simulink library "motohawk_engine_lib"  (Simulink 6.3)
undefined symbols (not defined in the file or in its folder): cast_val, IndPowerMax, InjSequence, lookup_group, MAF_Sensor_p, motohawk_tex, motohawk_vardec_config_group, motohawk_vardec_path, SampleTime, SparkSequence, SteadyStateECT, txtTitle, WarmUpTimeConst
libraries: MotoHawk_lib x234, motohawk_annotations_lib x22, motohawk_control_primitives_lib x20, motohawk_engine_lib x8, motohawk_control_primitives_lib_new x3
(part 5 of 7)

== system motohawk_engine_lib/PWM Characterization ==
  note: The outputs of this block are designed to be
      | directly connected to a MotoHawk PWM block.
  EngUnits : Inport
  Convert to integer 0.01Hz resolution : Gain  Gain=100  SaturateOnIntegerOverflow=on
  Convert to integer 14-bit PWM resolution : Gain  Gain=40.95  SaturateOnIntegerOverflow=on
  Data Type Conversion1 : DataTypeConversion  SaturateOnIntegerOverflow=on  RndMeth=Zero
  Data Type Conversion2 : DataTypeConversion  OutDataTypeMode=uint32  SaturateOnIntegerOverflow=on  RndMeth=Zero
  Data Type Conversion3 : DataTypeConversion  OutDataTypeMode=int16  SaturateOnIntegerOverflow=on  RndMeth=Zero
  Product : Product  SaturateOnIntegerOverflow=on  InputSameDT=on
  Saturation : motohawk_control_primitives_lib/Saturation
  Sum : Sum  Inputs=|++  SaturateOnIntegerOverflow=on
  motohawk_calibration : MotoHawk_lib/Calibration & Probing Blocks/motohawk_calibration  nam=[prefix 'Gain']  val=1  storage=Calibration  show_more=on  name_source=Use Parameter  data_type=double  read_level=1  write_level=1  ovr_cals=on  view_as=Number  enum_struct={'Disabled', 'Enabled'}  vector_style=Wide Row  use_help_units=on  help='Scaling from engineering units to PWM duty cycle'  units=['%/' units]  use_header_enum=off  row_header_enum={}  col_header_enum={}  use_min_max=off  min_val=-inf  max_val=inf  use_precision=off  precision=''  gain=1  offset=0  exp=1  use_mototune_group=on  mototune_group=[group ' | ' nam ' Config']
  motohawk_calibration1 : MotoHawk_lib/Calibration & Probing Blocks/motohawk_calibration  nam=[prefix 'Offset']  val=0  storage=Calibration  show_more=on  name_source=Use Parameter  data_type=double  read_level=1  write_level=1  ovr_cals=on  view_as=Number  enum_struct={'Disabled', 'Enabled'}  vector_style=Wide Row  use_help_units=on  help='Offset from engineering units to PWM duty cycle'  units='%'  use_header_enum=off  row_header_enum={}  col_header_enum={}  use_min_max=off  min_val=-inf  max_val=inf  use_precision=off  precision=''  gain=1  offset=0  exp=1  use_mototune_group=on  mototune_group=[group ' | ' nam ' Config']
  motohawk_calibration2 : MotoHawk_lib/Calibration & Probing Blocks/motohawk_calibration  nam=[prefix 'MinLimit']  val=0  storage=Calibration  show_more=on  name_source=Use Parameter  data_type=double  read_level=1  write_level=1  ovr_cals=on  view_as=Number  enum_struct={'Disabled', 'Enabled'}  vector_style=Wide Row  use_help_units=on  help='Minimum limit of PWM signal.'  units='%'  use_header_enum=off  row_header_enum={}  col_header_enum={}  use_min_max=off  min_val=-inf  max_val=inf  use_precision=off  precision=''  gain=1  offset=0  exp=1  use_mototune_group=on  mototune_group=[group ' | ' nam ' Config']
  motohawk_calibration3 : MotoHawk_lib/Calibration & Probing Blocks/motohawk_calibration  nam=[prefix 'MaxLimit']  val=100  storage=Calibration  show_more=on  name_source=Use Parameter  data_type=double  read_level=1  write_level=1  ovr_cals=on  view_as=Number  enum_struct={'Disabled', 'Enabled'}  vector_style=Wide Row  use_help_units=on  help='Maximum limit of PWM signal.'  units='%'  use_header_enum=off  row_header_enum={}  col_header_enum={}  use_min_max=off  min_val=-inf  max_val=inf  use_precision=off  precision=''  gain=1  offset=0  exp=1  use_mototune_group=on  mototune_group=[group ' | ' nam ' Config']
  motohawk_calibration4 : MotoHawk_lib/Calibration & Probing Blocks/motohawk_calibration  nam=[prefix 'Frequency']  val=100  storage=Calibration  show_more=on  name_source=Use Parameter  data_type=double  read_level=1  write_level=1  ovr_cals=on  view_as=Number  enum_struct={'Disabled', 'Enabled'}  vector_style=Wide Row  use_help_units=on  help='Frequency of PWM output'  units='Hz'  use_header_enum=off  row_header_enum={}  col_header_enum={}  use_min_max=off  min_val=-inf  max_val=inf  use_precision=off  precision=''  gain=1  offset=0  exp=1  use_mototune_group=on  mototune_group=[group ' | ' nam ' Config']
  motohawk_override_abs2 : MotoHawk_lib/Calibration & Probing Blocks/motohawk_override_abs  parent_name=nam  show_more=on  name_source=Use Parameter  parent_read_level=1  parent_override_level=1  view_as=Number  enum_struct={'Disabled', 'Enabled'}  use_help_units=on  parent_help='Override result of linear sensor characterization, in engineering units'  parent_units=units  use_min_max=on  parent_min=-inf  parent_max=inf  use_precision=off  parent_precision=''  parent_gain=1  parent_offset=0  parent_exp=1  use_mototune_group=on  parent_group=group
  motohawk_probe2 : MotoHawk_lib/Calibration & Probing Blocks/motohawk_probe  nam=[prefix 'DutyCycle']  show_more=on  name_source=Use Parameter  read_level=1  view_as=Number  enum_struct={'Disabled', 'Enabled'}  vector_style=Wide Row  use_help_units=on  help='Actual duty cycle of actuator'  units='%'  use_header_enum=off  row_header_enum={}  col_header_enum={}  use_precision=off  precision=''  gain=1  offset=0  exp=1  use_mototune_group=on  mototune_group=group
  DutyCycle : Outport
  Frequency : Outport  Port=2
  wires:
  Data Type Conversion2/1 -> Frequency/1
  Convert to integer 0.01Hz resolution/1 -> Data Type Conversion2/1
  motohawk_calibration4/1 -> Convert to integer 0.01Hz resolution/1
  Data Type Conversion1/1 -> Product/1
  motohawk_override_abs2/1 -> Data Type Conversion1/1
  EngUnits/1 -> motohawk_override_abs2/1
  Product/1 -> Sum/1
  motohawk_calibration1/1 -> Sum/2
  motohawk_calibration/1 -> Product/2
  Data Type Conversion3/1 -> DutyCycle/1
  Convert to integer 14-bit PWM resolution/1 -> Data Type Conversion3/1
  Sum/1 -> Saturation/1
  Saturation/1 -> Convert to integer 14-bit PWM resolution/1, motohawk_probe2/1
  motohawk_calibration2/1 -> Saturation/2
  motohawk_calibration3/1 -> Saturation/3

== system motohawk_engine_lib/Spark Coil Characterization ==
  SparkEnergy [mJ] : Inport
  SysVolt10Idx : Inport  Port=2
  Constant : Constant  Value=1000
  Constant1 : Constant  Value=0
  Only Enable Spark when Energy is Above Zero : RelationalOperator  Operator=>  ZeroCross=off  InputSameDT=on
  Product : Product  Inputs=*/  SaturateOnIntegerOverflow=on
  Sum : Sum  Inputs=|++  SaturateOnIntegerOverflow=on
  motohawk_TitleBlock : motohawk_annotations_lib/motohawk_TitleBlock  BlockType_='Mototron_Title_Block'  ttl='Spark Coil Characterization\newline\rmCalculations for spark coil dwell time vs. desired spark energy'  copyright="'THE INFORMATION CONTAINED IN THIS\\newlineDRAWING IS THE SOLE PROPERTY OF\\newlineMOTOTRON.  ANY REPRODUCTION IN\\newline PART OR AS A WHOLE WITHOUT THE\\newlineWRITTEN PERMISSION OF MOTOTRON\\newline IS PROHIBITED.\\fontsize{16}\\rm\\copyright\\rm\\fontsize{10} 2005'"  address='\fontsize{22}\it\fontname{Arial Black}MotoTron Corporation \fontname{Arial}\fontsize{10}\newline505 Marion Road, Oshkosh, WI, 54901\newlinewww.mototron.com (734) 822-7700'  image_file='mh.jpg'  pretty_print=on  edit_text=[motohawk_tex(get_param(bdroot, 'Description')) '\rm\newline' motohawk_tex(get_param(gcs, 'Name'))]  edit_as=6
  motohawk_calibration : MotoHawk_lib/Calibration & Probing Blocks/motohawk_calibration  nam='CoilDrvrDlyTime'  val=CoilDrvrDlyTime  storage=Calibration  show_more=on  name_source=Use Parameter  data_type=Inherit from 'Default Value'  read_level=1  write_level=1  ovr_cals=on  view_as=Number  enum_struct={'Disabled', 'Enabled'}  vector_style=Wide Row  use_help_units=on  help='Spark Coil Driver Delay Time'  units='us'  use_header_enum=off  row_header_enum={}  col_header_enum={}  use_min_max=off  min_val=-inf  max_val=inf  use_precision=off  precision=''  gain=1  offset=0  exp=1  use_mototune_group=off  mototune_group=lookup_group(gcb, 'CoilDrvrDlyTime')
  motohawk_interpolation_2d : MotoHawk_lib/Lookup Tables/motohawk_interpolation_2d  nam='CoilDwell'  table_data=CoilDwellMap  show_more=on  data_type=Inherit from 'Table Data'  storage=NonAdaptive  read_level=1  write_level=1  ovr_cals=on  use_help=on  help='Spark dwell time'  units='ms'  use_min_max=off  min_val=-inf  max_val=inf  use_precision=off  precision=''  gain=1  offset=0  exp=1  use_links=on  row_prelookup_block=''  col_prelookup_block=''  output_name='CoilDwell'  use_mototune_group=off  mototune_group=lookup_group(gcb, 'CoilDwell')
  motohawk_prelookup1 : MotoHawk_lib/Lookup Tables/motohawk_prelookup  nam='SpkEnergy10'  breakpoint_data=SpkEnergy10IdxArr  show_more=on  data_type=Inherit from 'Table Data'  storage=Constant  read_level=1  write_level=1  ovr_cals=on  use_help=on  help='Prelookup for Spark Energy'  units='mJ'  use_min_max=off  min_val=-inf  max_val=inf  use_precision=off  precision=''  gain=1  offset=0  exp=1  use_links=on  input_name='SparkEnergy'  use_mototune_group=off  mototune_group=lookup_group(gcb, 'SpkEnergy10')
  motohawk_probe : MotoHawk_lib/Calibration & Probing Blocks/motohawk_probe  nam='CoilDwell'  show_more=on  name_source=Use Parameter  read_level=1  view_as=Number  enum_struct={'Disabled', 'Enabled'}  vector_style=Wide Row  use_help_units=on  help='Total electrical spark dwell time'  units='ms'  use_header_enum=off  row_header_enum={}  col_header_enum={}  use_precision=off  precision=''  gain=1  offset=0  exp=1  use_mototune_group=off  mototune_group=lookup_group(gcb, 'CoilDwell')
  motohawk_probe1 : MotoHawk_lib/Calibration & Probing Blocks/motohawk_probe  nam='SparkEnergy'  show_more=on  name_source=Use Parameter  read_level=1  view_as=Number  enum_struct={'Disabled', 'Enabled'}  vector_style=Wide Row  use_help_units=on  help='Commanded spark energy, before conversion to dwell time'  units='mJ'  use_header_enum=off  row_header_enum={}  col_header_enum={}  use_precision=off  precision=''  gain=1  offset=0  exp=1  use_mototune_group=off  mototune_group=lookup_group(gcb, 'SparkEnergy')
  SparkDwell [ms] : Outport
  SparkEnable [bool] : Outport  Port=2
  wires:
  Constant1/1 -> Only Enable Spark when Energy is Above Zero/2
  Only Enable Spark when Energy is Above Zero/1 -> SparkEnable [bool]/1
  Constant/1 -> Product/2
  Product/1 -> Sum/2
  motohawk_calibration/1 -> Product/1
  motohawk_interpolation_2d/1 -> Sum/1
  Sum/1 -> SparkDwell [ms]/1, motohawk_probe/1
  SparkEnergy [mJ]/1 -> Only Enable Spark when Energy is Above Zero/1, motohawk_probe1/1, motohawk_prelookup1/1
  motohawk_prelookup1/1 -> motohawk_interpolation_2d/1  "SpkEnergy10Idx"
  SysVolt10Idx/1 -> motohawk_interpolation_2d/2  "SysVolt10Idx"

== system motohawk_engine_lib/Spark Coil Output ==
  SparkEnable : Inport
  SparkStartAngle [degCA] : Inport  Port=2
  SparkStopAngle [degCA] : Inport  Port=3
  CylEnable : Inport  Port=4
  Data Type Conversion : DataTypeConversion  SaturateOnIntegerOverflow=on  RndMeth=Zero
  Data Type Conversion1 : DataTypeConversion  SaturateOnIntegerOverflow=on  RndMeth=Zero
  Data Type Conversion2 : DataTypeConversion  SaturateOnIntegerOverflow=on  RndMeth=Zero
  Gain1 : Gain  Gain=16  SaturateOnIntegerOverflow=on
  Gain2 : Gain  Gain=16  SaturateOnIntegerOverflow=on
  Logical Operator : Logic  AllPortsSameDT=off
  motohawk_seq_out_est : MotoHawk_lib/Advanced Digital I//O/motohawk_seq_out_est  text_resource=EST 1  code_resource=RES_EST1  val_resource=-1  target=ECU555_80  resource_enum_str=(None)=-1,EST 1=36,EST 2=37,EST 3=38,EST 4=39,EST 5=40,EST 6=41,EST 7=42,EST 8=43,EST 9=44,EST 10=45,EST 11=46,EST 12=47,EST 13=48,EST 14=49,EST 15=50,EST 16=51  pulse_number=0  pulse_angle_offset=offset  stop_mode=Angle Controlled  update_mode=OS  granularity=Fine  use_max_duration=off  use_vardec=off  nam='EST'  read_level=1  write_level=1  group='System | I/O Pins | Outputs Config'
  wires:
  Gain2/1 -> Data Type Conversion1/1
  Gain1/1 -> Data Type Conversion2/1
  SparkStartAngle [degCA]/1 -> Gain2/1
  SparkStopAngle [degCA]/1 -> Gain1/1
  Data Type Conversion/1 -> motohawk_seq_out_est/1
  Data Type Conversion1/1 -> motohawk_seq_out_est/2
  Data Type Conversion2/1 -> motohawk_seq_out_est/3
  Logical Operator/1 -> Data Type Conversion/1
  SparkEnable/1 -> Logical Operator/2
  CylEnable/1 -> Logical Operator/1

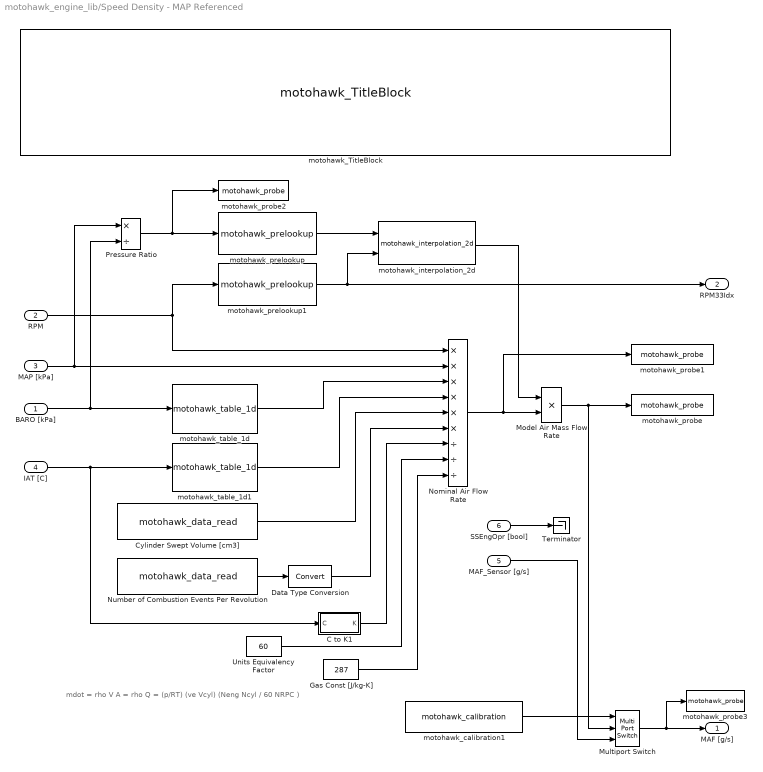
== system motohawk_engine_lib/Speed Density - MAP Referenced ==
  note: mdot = rho V A = rho Q = (p/RT) (ve Vcyl) (Neng Ncyl / 60 NRPC )
  BARO [kPa] : Inport
  RPM : Inport  Port=2
  MAP [kPa] : Inport  Port=3
  IAT [C] : Inport  Port=4
  MAF_Sensor [g/s] : Inport  Port=5
  SSEngOpr [bool] : Inport  Port=6
  C to K1 : Subsystem
      mask Display: disp('to')
  Cylinder Swept Volume [cm3] : MotoHawk_lib/Data Storage Blocks/motohawk_data_read  source=Lookup By Name  structure=Scalar  operation=Read scalar from location by index  sz_vec=-1  sz_row=-1  sz_col=-1  typ=double  nam='CylSweptVol'  checkNull=on  struct_inst_name='Struct1'
  Data Type Conversion : DataTypeConversion  SaturateOnIntegerOverflow=on  RndMeth=Zero
  Gas Const [J/kg-K] : Constant  Value=287
  Model Air Mass Flow Rate : Product  Inputs=**  SaturateOnIntegerOverflow=on  InputSameDT=on
  Multiport Switch : MultiPortSwitch  Inputs=2  zeroidx=on  SaturateOnIntegerOverflow=on  InputSameDT=on
  Nominal Air Flow Rate : Product  Inputs=******///  SaturateOnIntegerOverflow=on  InputSameDT=on
  Number of Combustion Events Per Revolution : MotoHawk_lib/Data Storage Blocks/motohawk_data_read  source=Lookup By Name  structure=Scalar  operation=Read scalar from location by index  sz_vec=-1  sz_row=-1  sz_col=-1  typ=uint8  nam='CombEventsPerRev'  checkNull=on  struct_inst_name='Struct1'
  Pressure Ratio : Product  Inputs=*/  SaturateOnIntegerOverflow=on  InputSameDT=on
  Terminator : Terminator
  Units Equivalency Factor : Constant  Value=60
  motohawk_TitleBlock : motohawk_annotations_lib/motohawk_TitleBlock  BlockType_='Mototron_Title_Block'  ttl='Compute Mass Airflow from Manifold Pressure and Temperature\newline\rmUses a Volumetric Efficiency map to adjust the results of the ideal gas law.'  copyright="'THE INFORMATION CONTAINED IN THIS\\newlineDRAWING IS THE SOLE PROPERTY OF\\newlineMOTOTRON.  ANY REPRODUCTION IN\\newline PART OR AS A WHOLE WITHOUT THE\\newlineWRITTEN PERMISSION OF MOTOTRON\\newline IS PROHIBITED.\\fontsize{16}\\rm\\copyright\\rm\\fontsize{10} 2005'"  address='\fontsize{22}\it\fontname{Arial Black}MotoTron Corporation \fontname{Arial}\fontsize{10}\newline505 Marion Road, Oshkosh, WI, 54901\newlinewww.mototron.com (734) 822-7700'  image_file='mh.jpg'  pretty_print=on  edit_text=[motohawk_tex(get_param(bdroot, 'Description')) '\rm\newline' motohawk_tex(get_param(gcs, 'Name'))]  edit_as=6
  motohawk_calibration1 : MotoHawk_lib/Calibration & Probing Blocks/motohawk_calibration  nam='MAF_Source'  val=MAF_Source  storage=Calibration  show_more=on  name_source=Use Parameter  data_type=uint8  read_level=1  write_level=1  ovr_cals=on  view_as=Enumeration  enum_struct={'Model from MAP', 'Use MAF sensor directly'}  vector_style=Wide Row  use_help_units=on  help='Selects the source for the fueling algorithm'  units=''  use_header_enum=off  row_header_enum={}  col_header_enum={}  use_min_max=off  min_val=-inf  max_val=inf  use_precision=off  precision=''  gain=1  offset=0  exp=1  use_mototune_group=on  mototune_group=lookup_group(gcb)
  motohawk_interpolation_2d : MotoHawk_lib/Lookup Tables/motohawk_interpolation_2d  nam='VolEff'  table_data=VolEffMap  show_more=on  data_type=Inherit from 'Table Data'  storage=NonAdaptive  read_level=1  write_level=1  ovr_cals=on  use_help=on  help='Volumetric Efficiency'  units='mult'  use_min_max=off  min_val=-inf  max_val=inf  use_precision=on  precision='6.4'  gain=1  offset=0  exp=1  use_links=off  row_prelookup_block=''  col_prelookup_block=''  output_name=''  use_mototune_group=on  mototune_group=lookup_group(gcb)
  motohawk_prelookup : MotoHawk_lib/Lookup Tables/motohawk_prelookup  nam='PressRatio17'  breakpoint_data=PressRatio17IdxArr  show_more=on  data_type=Inherit from 'Table Data'  storage=Constant  read_level=1  write_level=1  ovr_cals=on  use_help=on  help='Prelookup for Pressure Ratio'  units='ratio'  use_min_max=off  min_val=-inf  max_val=inf  use_precision=off  precision=''  gain=1  offset=0  exp=1  use_links=on  input_name='PressRatio'  use_mototune_group=on  mototune_group=lookup_group(gcb)
  motohawk_prelookup1 : MotoHawk_lib/Lookup Tables/motohawk_prelookup  nam='RPM17'  breakpoint_data=RPM17IdxArr  show_more=on  data_type=Inherit from 'Table Data'  storage=Constant  read_level=1  write_level=1  ovr_cals=on  use_help=on  help='Prelookup for RPM'  units='RPM'  use_min_max=off  min_val=-inf  max_val=inf  use_precision=off  precision=''  gain=1  offset=0  exp=1  use_links=on  input_name='RPM'  use_mototune_group=on  mototune_group=lookup_group(gcb)
  motohawk_probe : MotoHawk_lib/Calibration & Probing Blocks/motohawk_probe  nam='MAF_Model'  show_more=on  name_source=Use Parameter  read_level=1  view_as=Number  enum_struct={'Disabled', 'Enabled'}  vector_style=Wide Row  use_help_units=on  help='Air Mass Flow Rate - Port Total'  units='g/s'  use_header_enum=off  row_header_enum={}  col_header_enum={}  use_precision=off  precision=''  gain=1  offset=0  exp=1  use_mototune_group=on  mototune_group=lookup_group(gcb)
  motohawk_probe1 : MotoHawk_lib/Calibration & Probing Blocks/motohawk_probe  nam='MAF_Ideal'  show_more=on  name_source=Use Parameter  read_level=1  view_as=Number  enum_struct={'Disabled', 'Enabled'}  vector_style=Wide Row  use_help_units=on  help='Air Mass Flow Rate - ideal'  units='g/s'  use_header_enum=off  row_header_enum={}  col_header_enum={}  use_precision=off  precision=''  gain=1  offset=0  exp=1  use_mototune_group=on  mototune_group=lookup_group(gcb)
  motohawk_probe2 : MotoHawk_lib/Calibration & Probing Blocks/motohawk_probe  nam='PressRatio'  show_more=on  name_source=Use Parameter  read_level=1  view_as=Number  enum_struct={'Disabled', 'Enabled'}  vector_style=Wide Row  use_help_units=on  help='Pressure ratio - MAP over BARO'  units='ratio'  use_header_enum=off  row_header_enum={}  col_header_enum={}  use_precision=off  precision=''  gain=1  offset=0  exp=1  use_mototune_group=on  mototune_group=lookup_group(gcb)
  motohawk_probe3 : MotoHawk_lib/Calibration & Probing Blocks/motohawk_probe  nam='MAF'  show_more=on  name_source=Use Parameter  read_level=1  view_as=Number  enum_struct={'Disabled', 'Enabled'}  vector_style=Wide Row  use_help_units=on  help='Air mass flow rate at the intake manifold - Used by the fueling algorithm'  units='g/s'  use_header_enum=off  row_header_enum={}  col_header_enum={}  use_precision=off  precision=''  gain=1  offset=0  exp=1  use_mototune_group=on  mototune_group=lookup_group(gcb)
  motohawk_table_1d : MotoHawk_lib/Lookup Tables/motohawk_table_1d  nam='VEPressCorr'  bp_nam='BARO17'  breakpoint_data=BARO17IdxArr  table_data=VEPressCorrTbl  show_more=on  bp_data_type=Inherit from 'Breakpoint Data'  table_data_type=Inherit from 'Table Data'  storage=NonAdaptive  read_level=1  write_level=1  ovr_cals=on  use_help=off  help=''  bp_units=''  table_units=''  use_min_max=off  bp_min_val=-inf  bp_max_val=inf  min_val=-inf  max_val=inf  use_precision=off  use_breakpoint=off  b_precision=''  b_gain=1  b_offset=0  b_exp=1  use_table=off  t_precision=''  t_gain=1  t_offset=0  t_exp=1  use_links=on  input_name='BARO'  output_name=''  use_mototune_group=on  mototune_group=lookup_group(gcb)
  motohawk_table_1d1 : MotoHawk_lib/Lookup Tables/motohawk_table_1d  nam='VETempCorr'  bp_nam='IAT17'  breakpoint_data=IAT17IdxArr  table_data=VETempCorrTbl  show_more=on  bp_data_type=Inherit from 'Breakpoint Data'  table_data_type=Inherit from 'Table Data'  storage=NonAdaptive  read_level=1  write_level=1  ovr_cals=on  use_help=off  help=''  bp_units=''  table_units=''  use_min_max=off  bp_min_val=-inf  bp_max_val=inf  min_val=-inf  max_val=inf  use_precision=off  use_breakpoint=off  b_precision=''  b_gain=1  b_offset=0  b_exp=1  use_table=off  t_precision=''  t_gain=1  t_offset=0  t_exp=1  use_links=on  input_name='IAT'  output_name=''  use_mototune_group=on  mototune_group=lookup_group(gcb)
  MAF [g/s] : Outport
  RPM33Idx : Outport  Port=2
  wires:
  SSEngOpr [bool]/1 -> Terminator/1
  Data Type Conversion/1 -> Nominal Air Flow Rate/6
  Nominal Air Flow Rate/1 -> motohawk_probe1/1, Model Air Mass Flow Rate/2
  Gas Const [J/kg-K]/1 -> Nominal Air Flow Rate/9
  Units Equivalency Factor/1 -> Nominal Air Flow Rate/8
  C to K1/1(K) -> Nominal Air Flow Rate/7
  Number of Combustion Events Per Revolution/1 -> Data Type Conversion/1
  Cylinder Swept Volume [cm3]/1 -> Nominal Air Flow Rate/5
  motohawk_table_1d1/1 -> Nominal Air Flow Rate/4
  motohawk_table_1d/1 -> Nominal Air Flow Rate/3
  MAP [kPa]/1 -> Nominal Air Flow Rate/2, Pressure Ratio/1
  BARO [kPa]/1 -> motohawk_table_1d/1, Pressure Ratio/2
  RPM/1 -> motohawk_prelookup1/1, Nominal Air Flow Rate/1
  IAT [C]/1 -> motohawk_table_1d1/1, C to K1/1(C)
  Pressure Ratio/1 -> motohawk_probe2/1, motohawk_prelookup/1
  Model Air Mass Flow Rate/1 -> Multiport Switch/2, motohawk_probe/1
  motohawk_interpolation_2d/1 -> Model Air Mass Flow Rate/1
  motohawk_prelookup/1 -> motohawk_interpolation_2d/1
  motohawk_prelookup1/1 -> motohawk_interpolation_2d/2, RPM33Idx/1
  MAF_Sensor [g/s]/1 -> Multiport Switch/3
  Multiport Switch/1 -> MAF [g/s]/1, motohawk_probe3/1
  motohawk_calibration1/1 -> Multiport Switch/1

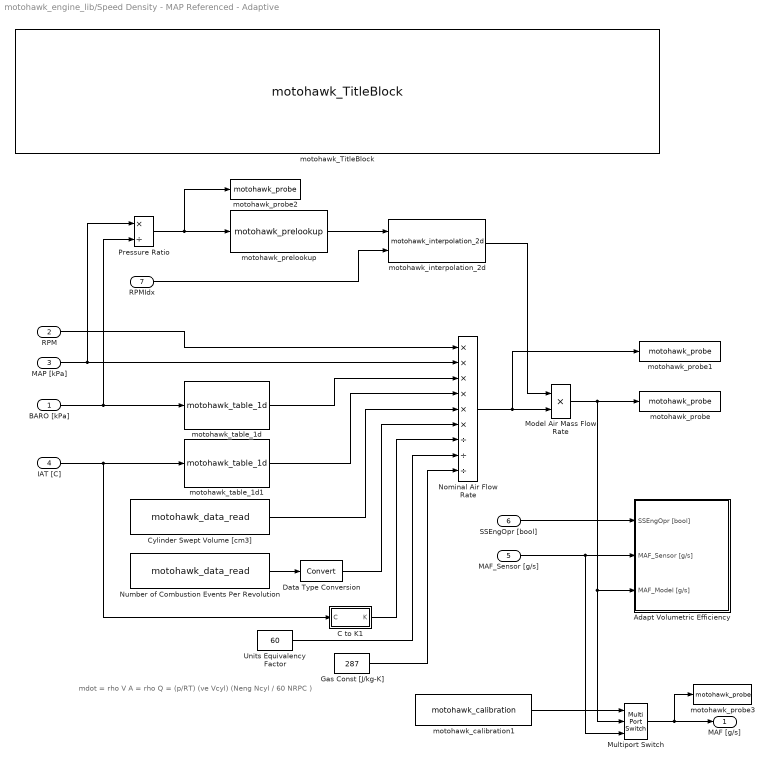
== system motohawk_engine_lib/Speed Density - MAP Referenced - Adaptive ==
  note: mdot = rho V A = rho Q = (p/RT) (ve Vcyl) (Neng Ncyl / 60 NRPC )
  BARO [kPa] : Inport
  RPM : Inport  Port=2
  MAP [kPa] : Inport  Port=3
  IAT [C] : Inport  Port=4
  MAF_Sensor [g/s] : Inport  Port=5
  SSEngOpr [bool] : Inport  Port=6
  RPMIdx : Inport  Port=7
  Adapt Volumetric Efficiency : Subsystem
  C to K1 : Subsystem
      mask Display: disp('to')
  Cylinder Swept Volume [cm3] : MotoHawk_lib/Data Storage Blocks/motohawk_data_read  source=Lookup By Name  structure=Scalar  operation=Read scalar from location by index  sz_vec=-1  sz_row=-1  sz_col=-1  typ=double  nam='CylSweptVol'  checkNull=on  struct_inst_name='Struct1'
  Data Type Conversion : DataTypeConversion  SaturateOnIntegerOverflow=on  RndMeth=Zero
  Gas Const [J/kg-K] : Constant  Value=287
  Model Air Mass Flow Rate : Product  Inputs=**  SaturateOnIntegerOverflow=on  InputSameDT=on
  Multiport Switch : MultiPortSwitch  Inputs=2  zeroidx=on  SaturateOnIntegerOverflow=on  InputSameDT=on
  Nominal Air Flow Rate : Product  Inputs=******///  SaturateOnIntegerOverflow=on  InputSameDT=on
  Number of Combustion Events Per Revolution : MotoHawk_lib/Data Storage Blocks/motohawk_data_read  source=Lookup By Name  structure=Scalar  operation=Read scalar from location by index  sz_vec=-1  sz_row=-1  sz_col=-1  typ=uint8  nam='CombEventsPerRev'  checkNull=on  struct_inst_name='Struct1'
  Pressure Ratio : Product  Inputs=*/  SaturateOnIntegerOverflow=on  InputSameDT=on
  Units Equivalency Factor : Constant  Value=60
  motohawk_TitleBlock : motohawk_annotations_lib/motohawk_TitleBlock  BlockType_='Mototron_Title_Block'  ttl='Compute Mass Airflow from Manifold Pressure and Temperature\newline\rmUses a Volumetric Efficiency map to adjust the results of the ideal gas law.'  copyright="'THE INFORMATION CONTAINED IN THIS\\newlineDRAWING IS THE SOLE PROPERTY OF\\newlineMOTOTRON.  ANY REPRODUCTION IN\\newline PART OR AS A WHOLE WITHOUT THE\\newlineWRITTEN PERMISSION OF MOTOTRON\\newline IS PROHIBITED.\\fontsize{16}\\rm\\copyright\\rm\\fontsize{10} 2005'"  address='\fontsize{22}\it\fontname{Arial Black}MotoTron Corporation \fontname{Arial}\fontsize{10}\newline505 Marion Road, Oshkosh, WI, 54901\newlinewww.mototron.com (734) 822-7700'  image_file='mh.jpg'  pretty_print=on  edit_text=[motohawk_tex(get_param(bdroot, 'Description')) '\rm\newline' motohawk_tex(get_param(gcs, 'Name'))]  edit_as=6
  motohawk_calibration1 : MotoHawk_lib/Calibration & Probing Blocks/motohawk_calibration  nam='MAF_Source'  val=0  storage=Display  show_more=on  name_source=Use Parameter  data_type=uint8  read_level=1  write_level=1  ovr_cals=on  view_as=Enumeration  enum_struct={'Model from MAP', 'Use MAF sensor directly'}  vector_style=Wide Row  use_help_units=on  help='Selects the source for the fueling algorithm'  units=''  use_header_enum=off  row_header_enum={}  col_header_enum={}  use_min_max=off  min_val=-inf  max_val=inf  use_precision=off  precision=''  gain=1  offset=0  exp=1  use_mototune_group=on  mototune_group=lookup_group(gcb)
  motohawk_interpolation_2d : MotoHawk_lib/Lookup Tables/motohawk_interpolation_2d  nam='VolEff'  table_data=VolEffMap  show_more=on  data_type=Inherit from 'Table Data'  storage=Adaptive - NonVolatile  read_level=1  write_level=1  ovr_cals=on  use_help=off  help='Volumetric Efficiency'  units='mult'  use_min_max=off  min_val=-inf  max_val=inf  use_precision=off  precision='5.3'  gain=1  offset=0  exp=1  use_links=off  row_prelookup_block=''  col_prelookup_block=''  output_name=''  use_mototune_group=off  mototune_group=lookup_group(gcb)
  motohawk_prelookup : MotoHawk_lib/Lookup Tables/motohawk_prelookup  nam='PressRatio17'  breakpoint_data=PressRatio17IdxArr  show_more=on  data_type=Inherit from 'Table Data'  storage=Constant  read_level=1  write_level=1  ovr_cals=on  use_help=on  help='Prelookup for Pressure Ratio'  units='ratio'  use_min_max=off  min_val=-inf  max_val=inf  use_precision=off  precision=''  gain=1  offset=0  exp=1  use_links=on  input_name='PressRatio'  use_mototune_group=on  mototune_group='Indexes'
  motohawk_probe : MotoHawk_lib/Calibration & Probing Blocks/motohawk_probe  nam='MAF_Model'  show_more=on  name_source=Use Parameter  read_level=1  view_as=Number  enum_struct={'Disabled', 'Enabled'}  vector_style=Wide Row  use_help_units=on  help='Air Mass Flow Rate - Port Total'  units='g/s'  use_header_enum=off  row_header_enum={}  col_header_enum={}  use_precision=off  precision=''  gain=1  offset=0  exp=1  use_mototune_group=on  mototune_group=lookup_group(gcb)
  motohawk_probe1 : MotoHawk_lib/Calibration & Probing Blocks/motohawk_probe  nam='MAF_Ideal'  show_more=on  name_source=Use Parameter  read_level=1  view_as=Number  enum_struct={'Disabled', 'Enabled'}  vector_style=Wide Row  use_help_units=on  help='Air Mass Flow Rate - ideal'  units='g/s'  use_header_enum=off  row_header_enum={}  col_header_enum={}  use_precision=off  precision=''  gain=1  offset=0  exp=1  use_mototune_group=on  mototune_group=lookup_group(gcb)
  motohawk_probe2 : MotoHawk_lib/Calibration & Probing Blocks/motohawk_probe  nam='PressRatio'  show_more=on  name_source=Use Parameter  read_level=1  view_as=Number  enum_struct={'Disabled', 'Enabled'}  vector_style=Wide Row  use_help_units=on  help='Pressure ratio - MAP over BARO'  units='ratio'  use_header_enum=off  row_header_enum={}  col_header_enum={}  use_precision=off  precision=''  gain=1  offset=0  exp=1  use_mototune_group=on  mototune_group=lookup_group(gcb)
  motohawk_probe3 : MotoHawk_lib/Calibration & Probing Blocks/motohawk_probe  nam='MAF'  show_more=on  name_source=Use Parameter  read_level=1  view_as=Number  enum_struct={'Disabled', 'Enabled'}  vector_style=Wide Row  use_help_units=on  help='Air mass flow rate at the intake manifold - Used by the fueling algorithm'  units='g/s'  use_header_enum=off  row_header_enum={}  col_header_enum={}  use_precision=off  precision=''  gain=1  offset=0  exp=1  use_mototune_group=on  mototune_group=lookup_group(gcb)
  motohawk_table_1d : MotoHawk_lib/Lookup Tables/motohawk_table_1d  nam='VEPressCorr'  bp_nam='BARO17'  breakpoint_data=BARO17IdxArr  table_data=VEPressCorrTbl  show_more=on  bp_data_type=Inherit from 'Breakpoint Data'  table_data_type=Inherit from 'Table Data'  storage=NonAdaptive  read_level=1  write_level=1  ovr_cals=on  use_help=off  help=''  bp_units=''  table_units=''  use_min_max=off  bp_min_val=-inf  bp_max_val=inf  min_val=-inf  max_val=inf  use_precision=off  use_breakpoint=off  b_precision=''  b_gain=1  b_offset=0  b_exp=1  use_table=off  t_precision=''  t_gain=1  t_offset=0  t_exp=1  use_links=on  input_name='BARO'  output_name=''  use_mototune_group=on  mototune_group=lookup_group(gcb)
  motohawk_table_1d1 : MotoHawk_lib/Lookup Tables/motohawk_table_1d  nam='VETempCorr'  bp_nam='IAT17'  breakpoint_data=IAT17IdxArr  table_data=VETempCorrTbl  show_more=on  bp_data_type=Inherit from 'Breakpoint Data'  table_data_type=Inherit from 'Table Data'  storage=NonAdaptive  read_level=1  write_level=1  ovr_cals=on  use_help=off  help=''  bp_units=''  table_units=''  use_min_max=off  bp_min_val=-inf  bp_max_val=inf  min_val=-inf  max_val=inf  use_precision=off  use_breakpoint=off  b_precision=''  b_gain=1  b_offset=0  b_exp=1  use_table=off  t_precision=''  t_gain=1  t_offset=0  t_exp=1  use_links=on  input_name='IAT'  output_name=''  use_mototune_group=on  mototune_group=lookup_group(gcb)
  MAF [g/s] : Outport
  wires:
  SSEngOpr [bool]/1 -> Adapt Volumetric Efficiency/1(SSEngOpr [bool])
  motohawk_calibration1/1 -> Multiport Switch/1
  Multiport Switch/1 -> motohawk_probe3/1, MAF [g/s]/1
  MAF_Sensor [g/s]/1 -> Adapt Volumetric Efficiency/2(MAF_Sensor [g/s]), Multiport Switch/3
  RPMIdx/1 -> motohawk_interpolation_2d/2
  motohawk_prelookup/1 -> motohawk_interpolation_2d/1
  motohawk_interpolation_2d/1 -> Model Air Mass Flow Rate/1
  Model Air Mass Flow Rate/1 -> Adapt Volumetric Efficiency/3(MAF_Model [g/s]), Multiport Switch/2, motohawk_probe/1
  Pressure Ratio/1 -> motohawk_prelookup/1, motohawk_probe2/1
  IAT [C]/1 -> C to K1/1(C), motohawk_table_1d1/1
  RPM/1 -> Nominal Air Flow Rate/1
  BARO [kPa]/1 -> Pressure Ratio/2, motohawk_table_1d/1
  MAP [kPa]/1 -> Pressure Ratio/1, Nominal Air Flow Rate/2
  motohawk_table_1d/1 -> Nominal Air Flow Rate/3
  motohawk_table_1d1/1 -> Nominal Air Flow Rate/4
  Cylinder Swept Volume [cm3]/1 -> Nominal Air Flow Rate/5
  Number of Combustion Events Per Revolution/1 -> Data Type Conversion/1
  C to K1/1(K) -> Nominal Air Flow Rate/7
  Units Equivalency Factor/1 -> Nominal Air Flow Rate/8
  Gas Const [J/kg-K]/1 -> Nominal Air Flow Rate/9
  Nominal Air Flow Rate/1 -> Model Air Mass Flow Rate/2, motohawk_probe1/1
  Data Type Conversion/1 -> Nominal Air Flow Rate/6

== system motohawk_engine_lib/Stop Angle to Start Angle ==
  Stop Angle [degCA] : Inport
  RPM : Inport  Port=2
  PulseWidth [ms] : Inport  Port=3
  Product1 : Product  Inputs=**/  SaturateOnIntegerOverflow=on  InputSameDT=on
  Product2 : Product  Inputs=**  SaturateOnIntegerOverflow=on  InputSameDT=on
  Sum : Sum  Inputs=|++  SaturateOnIntegerOverflow=on  InputSameDT=on
  deg/rev : Constant  Value=360
  min/msec : Constant  Value=60000
  motohawk_TitleBlock : motohawk_annotations_lib/motohawk_TitleBlock  BlockType_='Mototron_Title_Block'  ttl='Stop Angle to Start Angle Calculation\newline\rmConverts from EOI to SOI, for example, in degrees before TDC.'  copyright="'THE INFORMATION CONTAINED IN THIS\\newlineDRAWING IS THE SOLE PROPERTY OF\\newlineMOTOTRON.  ANY REPRODUCTION IN\\newline PART OR AS A WHOLE WITHOUT THE\\newlineWRITTEN PERMISSION OF MOTOTRON\\newline IS PROHIBITED.\\fontsize{16}\\rm\\copyright\\rm\\fontsize{10} 2005'"  address='\fontsize{22}\it\fontname{Arial Black}MotoTron Corporation \fontname{Arial}\fontsize{10}\newline505 Marion Road, Oshkosh, WI, 54901\newlinewww.mototron.com (734) 822-7700'  image_file='mh.jpg'  pretty_print=on  edit_text=[motohawk_tex(get_param(bdroot, 'Description')) '\rm\newline' motohawk_tex(get_param(gcs, 'Name'))]  edit_as=6
  Start Angle [degCA] : Outport
  wires:
  Product2/1 -> Sum/2  "PulseWidth [degCA]"
  Product1/1 -> Product2/1  "deg/ms"
  PulseWidth [ms]/1 -> Product2/2  "PulseWidth [ms]"
  deg/rev/1 -> Product1/2
  min/msec/1 -> Product1/3
  RPM/1 -> Product1/1
  Sum/1 -> Start Angle [degCA]/1
  Stop Angle [degCA]/1 -> Sum/1

== system motohawk_engine_lib/Subsystem ==
  Enabled Subsystem : Subsystem  TreatAsAtomicUnit=on
  motohawk_fault_properties : MotoHawk_lib/Fault Management Blocks/motohawk_fault_properties  source=Lookup By Name  nam=fltnam  use_id=on  use_mode=off  use_xlim=off  use_ylim=off  use_x=off  use_y=off
  motohawk_fault_status : MotoHawk_lib/Fault Management Blocks/motohawk_fault_status  source=Lookup By Name  nam=fltnam  status=Active
  State : Outport
  Code : Outport  Port=2
  wires:
  Enabled Subsystem/1(Out1) -> Code/1
  motohawk_fault_status/1 -> State/1, Enabled Subsystem/Enable
  motohawk_fault_properties/1 -> Enabled Subsystem/1(In1)

== system motohawk_engine_lib/Capture Signal At Startup/Collect Average ==
  note: Collect samples by summing,
      | and divide by the total, to obtain average
  Count : Inport
  Signal : Inport  Port=2
  Enable : EnablePort
  Data Type Conversion : DataTypeConversion  SaturateOnIntegerOverflow=on  RndMeth=Zero
  Product : Product  Inputs=/*
  Sum1 : Sum  Inputs=|++  InputSameDT=on
  Unit Delay1 : UnitDelay  Orientation=left  SampleTime=-1
  Captured_Signal : Outport
  wires:
  Data Type Conversion/1 -> Product/1
  Count/1 -> Data Type Conversion/1
  Product/1 -> Captured_Signal/1
  Signal/1 -> Sum1/1
  Sum1/1 -> Product/2, Unit Delay1/1
  Unit Delay1/1 -> Sum1/2

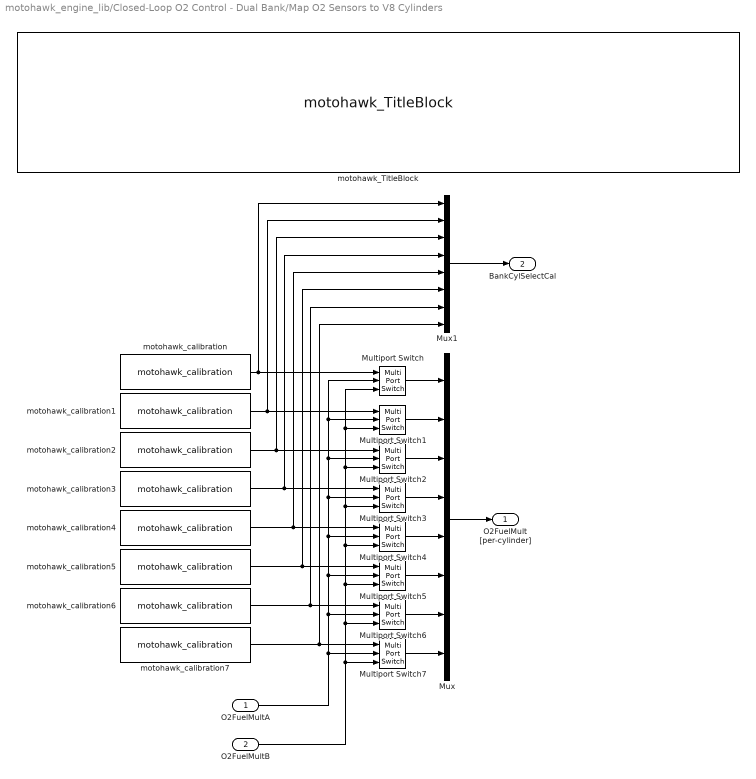
== system motohawk_engine_lib/Closed-Loop O2 Control - Dual Bank/Map O2 Sensors to V8 Cylinders ==
  O2FuelMultA : Inport
  O2FuelMultB : Inport  Port=2
  Multiport Switch{,1..7} (8 alike) : MultiPortSwitch  Inputs=2  zeroidx=on  InputSameDT=on
  Mux : Mux  Inputs=8
  Mux1 : Mux  Inputs=8
  motohawk_TitleBlock : motohawk_annotations_lib/motohawk_TitleBlock  BlockType_='Mototron_Title_Block'  ttl=[txtTitle '\newline\rmMapping from O2 Sensor Banks to Individual Cylinders']  copyright="'THE INFORMATION CONTAINED IN THIS\\newlineDRAWING IS THE SOLE PROPERTY OF\\newlineMOTOTRON.  ANY REPRODUCTION IN\\newline PART OR AS A WHOLE WITHOUT THE\\newlineWRITTEN PERMISSION OF MOTOTRON\\newline IS PROHIBITED.\\fontsize{16}\\rm\\copyright\\rm\\fontsize{10} 2005'"  address='\fontsize{22}\it\fontname{Arial Black}MotoTron Corporation \fontname{Arial}\fontsize{10}\newline505 Marion Road, Oshkosh, WI, 54901\newlinewww.mototron.com (734) 822-7700'  image_file='mh.jpg'  pretty_print=on  edit_text=[motohawk_tex(get_param(bdroot, 'Description')) '\rm\newline' motohawk_tex(get_param(gcs, 'Name'))]  edit_as=6
  motohawk_calibration : MotoHawk_lib/Calibration & Probing Blocks/motohawk_calibration  nam='O2Cyl1Select'  val=O2Cyl1Select  storage=Calibration  show_more=on  name_source=Use Parameter  data_type=uint8  read_level=1  write_level=1  ovr_cals=on  view_as=Enumeration  enum_struct={'O2A', 'O2B'}  vector_style=Wide Row  use_help_units=on  help='Select the O2 sensor mapped to cylinder 1'  units=''  use_header_enum=off  row_header_enum={}  col_header_enum={}  use_min_max=off  min_val=-inf  max_val=inf  use_precision=off  precision=''  gain=1  offset=0  exp=1  use_mototune_group=on  mototune_group=lookup_group(gcb, 'O2CylSelect')
  motohawk_calibration1 : MotoHawk_lib/Calibration & Probing Blocks/motohawk_calibration  nam='O2Cyl2Select'  val=O2Cyl2Select  storage=Calibration  show_more=on  name_source=Use Parameter  data_type=uint8  read_level=1  write_level=1  ovr_cals=on  view_as=Enumeration  enum_struct={'O2A', 'O2B'}  vector_style=Wide Row  use_help_units=on  help='Select the O2 sensor mapped to cylinder 2'  units=''  use_header_enum=off  row_header_enum={}  col_header_enum={}  use_min_max=off  min_val=-inf  max_val=inf  use_precision=off  precision=''  gain=1  offset=0  exp=1  use_mototune_group=on  mototune_group=lookup_group(gcb, 'O2CylSelect')
  motohawk_calibration2 : MotoHawk_lib/Calibration & Probing Blocks/motohawk_calibration  nam='O2Cyl3Select'  val=O2Cyl3Select  storage=Calibration  show_more=on  name_source=Use Parameter  data_type=uint8  read_level=1  write_level=1  ovr_cals=on  view_as=Enumeration  enum_struct={'O2A', 'O2B'}  vector_style=Wide Row  use_help_units=on  help='Select the O2 sensor mapped to cylinder 3'  units=''  use_header_enum=off  row_header_enum={}  col_header_enum={}  use_min_max=off  min_val=-inf  max_val=inf  use_precision=off  precision=''  gain=1  offset=0  exp=1  use_mototune_group=on  mototune_group=lookup_group(gcb, 'O2CylSelect')
  motohawk_calibration3 : MotoHawk_lib/Calibration & Probing Blocks/motohawk_calibration  nam='O2Cyl4Select'  val=O2Cyl4Select  storage=Calibration  show_more=on  name_source=Use Parameter  data_type=uint8  read_level=1  write_level=1  ovr_cals=on  view_as=Enumeration  enum_struct={'O2A', 'O2B'}  vector_style=Wide Row  use_help_units=on  help='Select the O2 sensor mapped to cylinder 4'  units=''  use_header_enum=off  row_header_enum={}  col_header_enum={}  use_min_max=off  min_val=-inf  max_val=inf  use_precision=off  precision=''  gain=1  offset=0  exp=1  use_mototune_group=on  mototune_group=lookup_group(gcb, 'O2CylSelect')
  motohawk_calibration4 : MotoHawk_lib/Calibration & Probing Blocks/motohawk_calibration  nam='O2Cyl5Select'  val=O2Cyl5Select  storage=Calibration  show_more=on  name_source=Use Parameter  data_type=uint8  read_level=1  write_level=1  ovr_cals=on  view_as=Enumeration  enum_struct={'O2A', 'O2B'}  vector_style=Wide Row  use_help_units=on  help='Select the O2 sensor mapped to cylinder 5'  units=''  use_header_enum=off  row_header_enum={}  col_header_enum={}  use_min_max=off  min_val=-inf  max_val=inf  use_precision=off  precision=''  gain=1  offset=0  exp=1  use_mototune_group=on  mototune_group=lookup_group(gcb, 'O2CylSelect')
  motohawk_calibration5 : MotoHawk_lib/Calibration & Probing Blocks/motohawk_calibration  nam='O2Cyl6Select'  val=O2Cyl6Select  storage=Calibration  show_more=on  name_source=Use Parameter  data_type=uint8  read_level=1  write_level=1  ovr_cals=on  view_as=Enumeration  enum_struct={'O2A', 'O2B'}  vector_style=Wide Row  use_help_units=on  help='Select the O2 sensor mapped to cylinder 6'  units=''  use_header_enum=off  row_header_enum={}  col_header_enum={}  use_min_max=off  min_val=-inf  max_val=inf  use_precision=off  precision=''  gain=1  offset=0  exp=1  use_mototune_group=on  mototune_group=lookup_group(gcb, 'O2CylSelect')
  motohawk_calibration6 : MotoHawk_lib/Calibration & Probing Blocks/motohawk_calibration  nam='O2Cyl7Select'  val=O2Cyl7Select  storage=Calibration  show_more=on  name_source=Use Parameter  data_type=uint8  read_level=1  write_level=1  ovr_cals=on  view_as=Enumeration  enum_struct={'O2A', 'O2B'}  vector_style=Wide Row  use_help_units=on  help='Select the O2 sensor mapped to cylinder 7'  units=''  use_header_enum=off  row_header_enum={}  col_header_enum={}  use_min_max=off  min_val=-inf  max_val=inf  use_precision=off  precision=''  gain=1  offset=0  exp=1  use_mototune_group=on  mototune_group=lookup_group(gcb, 'O2CylSelect')
  motohawk_calibration7 : MotoHawk_lib/Calibration & Probing Blocks/motohawk_calibration  nam='O2Cyl8Select'  val=O2Cyl8Select  storage=Calibration  show_more=on  name_source=Use Parameter  data_type=uint8  read_level=1  write_level=1  ovr_cals=on  view_as=Enumeration  enum_struct={'O2A', 'O2B'}  vector_style=Wide Row  use_help_units=on  help='Select the O2 sensor mapped to cylinder 8'  units=''  use_header_enum=off  row_header_enum={}  col_header_enum={}  use_min_max=off  min_val=-inf  max_val=inf  use_precision=off  precision=''  gain=1  offset=0  exp=1  use_mototune_group=on  mototune_group=lookup_group(gcb, 'O2CylSelect')
  O2FuelMult [per-cylinder] : Outport
  BankCylSelectCal : Outport  Port=2
  wires:
  motohawk_calibration/1 -> Multiport Switch/1, Mux1/1
  motohawk_calibration1/1 -> Multiport Switch1/1, Mux1/2
  motohawk_calibration2/1 -> Multiport Switch2/1, Mux1/3
  motohawk_calibration3/1 -> Multiport Switch3/1, Mux1/4
  motohawk_calibration4/1 -> Multiport Switch4/1, Mux1/5
  motohawk_calibration5/1 -> Multiport Switch5/1, Mux1/6
  motohawk_calibration6/1 -> Multiport Switch6/1, Mux1/7
  motohawk_calibration7/1 -> Multiport Switch7/1, Mux1/8
  O2FuelMultA/1 -> Multiport Switch/2, Multiport Switch1/2, Multiport Switch2/2, Multiport Switch3/2, Multiport Switch4/2, Multiport Switch5/2, Multiport Switch6/2, Multiport Switch7/2
  O2FuelMultB/1 -> Multiport Switch/3, Multiport Switch1/3, Multiport Switch2/3, Multiport Switch3/3, Multiport Switch4/3, Multiport Switch5/3, Multiport Switch6/3, Multiport Switch7/3
  Multiport Switch/1 -> Mux/1
  Multiport Switch1/1 -> Mux/2
  Multiport Switch2/1 -> Mux/3
  Multiport Switch3/1 -> Mux/4
  Multiport Switch4/1 -> Mux/5
  Multiport Switch5/1 -> Mux/6
  Multiport Switch6/1 -> Mux/7
  Multiport Switch7/1 -> Mux/8
  Mux/1 -> O2FuelMult [per-cylinder]/1
  Mux1/1 -> BankCylSelectCal/1

== system motohawk_engine_lib/Closed-Loop O2 Control - Dual Bank/O2 Control State Determination ==
  note: Closed-loop O2 control is disabled when running
      | enrichment or engine in ransient
  note: There are no O2 sensor faults
  note: Engine indicated work is above a threshold.
      | Usually a few minutes of idle time, to allow sensor warm-up.
  note: Desired equivalence ratio is within a delta of 1.0 (stoichiometric)
  O2ControlEnable [bool] : Inport
  DesEquivRatio : Inport  Port=2
  IndWork [kJ] : Inport  Port=3
  O2 Sensor Fault : Inport  Port=4
  Constant : Constant  OutDataTypeMode=single
  Logical Operator : Logic  AllPortsSameDT=off
  Logical Operator1 : Logic  Inputs=5
  Logical Operator3 : Logic  Operator=NOT  Inputs=3
  Relational Operator : RelationalOperator  Operator=<=  ZeroCross=off  InputSameDT=on
  Relational Operator1 : RelationalOperator  ZeroCross=off  InputSameDT=on
  Relational Operator2 : RelationalOperator  ZeroCross=off  InputSameDT=on
  Sum : Sum  Inputs=|++  SaturateOnIntegerOverflow=on
  Sum1 : Sum  Inputs=+-|  SaturateOnIntegerOverflow=on
  motohawk_TitleBlock : motohawk_annotations_lib/motohawk_TitleBlock  BlockType_='Mototron_Title_Block'  ttl=[txtTitle '\newline\rmClosed-Loop O2 Control State Determination']  copyright="'THE INFORMATION CONTAINED IN THIS\\newlineDRAWING IS THE SOLE PROPERTY OF\\newlineMOTOTRON.  ANY REPRODUCTION IN\\newline PART OR AS A WHOLE WITHOUT THE\\newlineWRITTEN PERMISSION OF MOTOTRON\\newline IS PROHIBITED.\\fontsize{16}\\rm\\copyright\\rm\\fontsize{10} 2005'"  address='\fontsize{22}\it\fontname{Arial Black}MotoTron Corporation \fontname{Arial}\fontsize{10}\newline505 Marion Road, Oshkosh, WI, 54901\newlinewww.mototron.com (734) 822-7700'  image_file='mh.jpg'  pretty_print=on  edit_text=[motohawk_tex(get_param(bdroot, 'Description')) '\rm\newline' motohawk_tex(get_param(gcs, 'Name'))]  edit_as=6
  motohawk_calibration : MotoHawk_lib/Calibration & Probing Blocks/motohawk_calibration  nam='O2ReadyIndWork'  val=O2ReadyIndWork  storage=Calibration  show_more=on  name_source=Use Parameter  data_type=Inherit from 'Default Value'  read_level=1  write_level=1  ovr_cals=on  view_as=Number  enum_struct={'Disabled', 'Enabled'}  vector_style=Wide Row  use_help_units=on  help='Minimum indicated work from engine before closed-loop O2 control will be enabled'  units='kJ'  use_header_enum=off  row_header_enum={}  col_header_enum={}  use_min_max=on  min_val=0  max_val=inf  use_precision=off  precision=''  gain=1  offset=0  exp=1  use_mototune_group=on  mototune_group=lookup_group(gcb, 'O2Config')
  motohawk_calibration1 : MotoHawk_lib/Calibration & Probing Blocks/motohawk_calibration  nam='O2EquivRatioDelta'  val=O2EquivRatioDelta  storage=Calibration  show_more=on  name_source=Use Parameter  data_type=Inherit from 'Default Value'  read_level=1  write_level=1  ovr_cals=on  view_as=Number  enum_struct={'Disabled', 'Enabled'}  vector_style=Wide Row  use_help_units=on  help='Equivalence ratio must be within this delta of stoichiometric to allow closed-loop O2 control'  units='ratio'  use_header_enum=off  row_header_enum={}  col_header_enum={}  use_min_max=on  min_val=0  max_val=1.0  use_precision=off  precision=''  gain=1  offset=0  exp=1  use_mototune_group=on  mototune_group=lookup_group(gcb, 'O2Config')
  motohawk_calibration2 : MotoHawk_lib/Calibration & Probing Blocks/motohawk_calibration  nam='O2ControlEnable'  val=O2ControlEnable  storage=Calibration  show_more=on  name_source=Use Parameter  data_type=boolean  read_level=1  write_level=1  ovr_cals=on  view_as=Enumeration  enum_struct={'Disabled', 'Enabled'}  vector_style=Wide Row  use_help_units=on  help='When enabled, the closed-loop O2 control algorithm is used'  units=''  use_header_enum=off  row_header_enum={}  col_header_enum={}  use_min_max=off  min_val=-inf  max_val=inf  use_precision=off  precision=''  gain=1  offset=0  exp=1  use_mototune_group=on  mototune_group=lookup_group(gcb, 'O2Config')
  motohawk_probe : MotoHawk_lib/Calibration & Probing Blocks/motohawk_probe  nam='O2Control'  show_more=on  name_source=Use Parameter  read_level=1  view_as=Enumeration  enum_struct={'Open-Loop', 'Closed-Loop'}  vector_style=Wide Row  use_help_units=on  help='Indicates whether closed-loop O2 control is currently enabled'  units=''  use_header_enum=off  row_header_enum={}  col_header_enum={}  use_precision=off  precision=''  gain=1  offset=0  exp=1  use_mototune_group=on  mototune_group=lookup_group(gcb, 'O2Display')
  O2Control : Outport
  wires:
  motohawk_calibration2/1 -> Logical Operator1/5
  O2ControlEnable [bool]/1 -> Logical Operator1/1
  Logical Operator1/1 -> motohawk_probe/1, O2Control/1
  motohawk_calibration1/1 -> Sum/1, Sum1/2
  Constant/1 -> Sum/2, Sum1/1
  DesEquivRatio/1 -> Relational Operator1/1, Relational Operator/1
  Sum/1 -> Relational Operator/2
  Sum1/1 -> Relational Operator1/2
  Relational Operator/1 -> Logical Operator/1
  Relational Operator1/1 -> Logical Operator/2
  IndWork [kJ]/1 -> Relational Operator2/1
  motohawk_calibration/1 -> Relational Operator2/2
  Relational Operator2/1 -> Logical Operator1/2
  Logical Operator/1 -> Logical Operator1/3
  O2 Sensor Fault/1 -> Logical Operator3/1
  Logical Operator3/1 -> Logical Operator1/4
